simulink model "SIS_VEZBA_4_SIMULINK_RESENO"  (R2018b)
settings: Solver=VariableStepAuto  StartTime=-0.1  StopTime=70  RelTol=1e-3
settings Model: Creator=Jovana  LastModifiedBy=Mieko

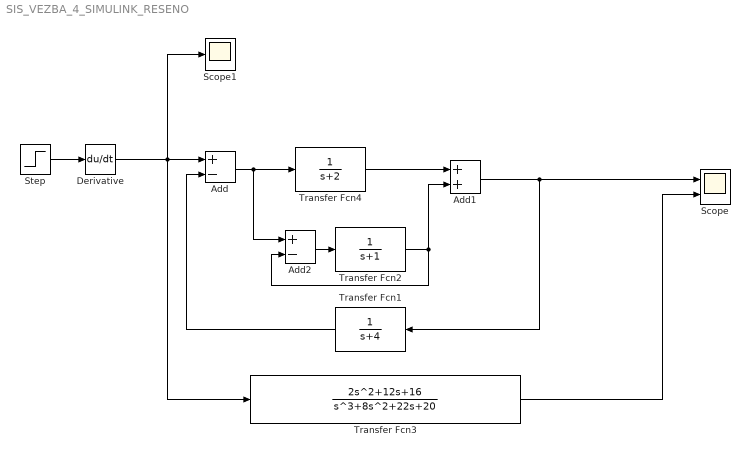
== system SIS_VEZBA_4_SIMULINK_RESENO ==
  Add : Sum  Inputs=+-
  Add1 : Sum
  Add2 : Sum  Inputs=+-
  Derivative : Derivative
  Scope : Scope  NumInputPorts=2
  Scope1 : Scope
  Step : Step  Time=0  SampleTime=0.01
  Transfer Fcn1 : TransferFcn  Denominator=[1 4]
  Transfer Fcn2 : TransferFcn  Denominator=[1 1]
  Transfer Fcn3 : TransferFcn  Numerator=[2 12 16]  Denominator=[1 8 22 20]
  Transfer Fcn4 : TransferFcn  Denominator=[1 2]
  wires:
  Step/1 -> Derivative/1
  Derivative/1 -> Transfer Fcn3/1, Add/1, Scope1/1
  Transfer Fcn3/1 -> Scope/2
  Add/1 -> Add2/1, Transfer Fcn4/1
  Transfer Fcn4/1 -> Add1/1
  Transfer Fcn1/1 -> Add/2
  Add1/1 -> Transfer Fcn1/1, Scope/1
  Transfer Fcn2/1 -> Add1/2, Add2/2
  Add2/1 -> Transfer Fcn2/1
